simulink library "WECSim_Lib"  (R2014b)
settings: Solver=ode45  StartTime=0.0  StopTime=10.0  RelTol=1e-3
undefined symbols (not defined in the file): body, constraint, pto, simu, waves, X, Y, Z
libraries: nesl_utility x107, sm_lib x53
(part 4 of 4)

== system WECSim_Lib/Body Elements/Rigid Body/Wave Diffraction and Excitation Force Calculation/Linear Wave Excitation Force Variant Subsystem/Regular Wave Excitation Force ==
  note: Calculates the wave force, F_wave, for the case of Regular Waves.
      |
      | F_wave =   A * cos(w * t) * Re{Fext}
      |                -  A * sin(w * t) * Im{Fext}
  In1 : Inport
  Add : Sum
  Add1 : Sum  Inputs=+-
  Constant : Constant  Value=pi/2
  Excitation Imaginary Part : Constant  Value=body.hydroForce.fExt.im(1,:)  VectorParams1D=off
  Excitation Real Part : Constant  Value=body.hydroForce.fExt.re(1,:)  VectorParams1D=off
  Product : Product
  Product1 : Product  Inputs=3
  Product2 : Product  Inputs=3
  Sine Wave Function : Sin  TimeSource=Use external signal  SampleTime=0
  Sine Wave Function1 : Sin  TimeSource=Use external signal  SampleTime=0
  Wave Amplitude : Constant  Value=waves.A(1,:)
  Wave Frequency : Constant  Value=waves.w(1,:)
  Out1 : Outport
  wires:
  In1/1 -> Product/1  "t"
  Wave Frequency/1 -> Product/2  "w"
  Product/1 -> Sine Wave Function/1, Add/1
  Sine Wave Function1/1 -> Product1/3  "cos(w*t)"
  Sine Wave Function/1 -> Product2/2  "sin(wt)"
  Excitation Imaginary Part/1 -> Product2/3  "Im{Fext}"
  Excitation Real Part/1 -> Product1/2  "Re{Fext}"
  Product1/1 -> Add1/1
  Product2/1 -> Add1/2
  Add1/1 -> Out1/1
  Wave Amplitude/1 -> Product2/1, Product1/1  "A"
  Add/1 -> Sine Wave Function1/1
  Constant/1 -> Add/2

== system WECSim_Lib/Body Elements/Rigid Body/Wave Diffraction and Excitation Force Calculation/Linear Wave Excitation Force Variant Subsystem/User Defined Wave Excitation Force ==
  note: Calculates the wave force, F_wave, for the case of User Defined Waves.
      |
      | F_wave = convulation calculation [1x6]
  InputWaveForceTimeHistory : FromWorkspace  VariableName=[waves.waveAmpTime(:,1),body.hydroForce.userDefinedFe]  SampleTime=0
  Out1 : Outport
  wires:
  InputWaveForceTimeHistory/1 -> Out1/1

== system WECSim_Lib/Body Elements/Rigid Body/Wave Diffraction and Excitation Force Calculation/Nonlinear FK Force Variant Subsystem/No Nonlinear FroudeKrylov Force ==
  Constant : Constant  Value=[0 0 0 0 0 0]
  Out1 : Outport
  wires:
  Constant/1 -> Out1/1

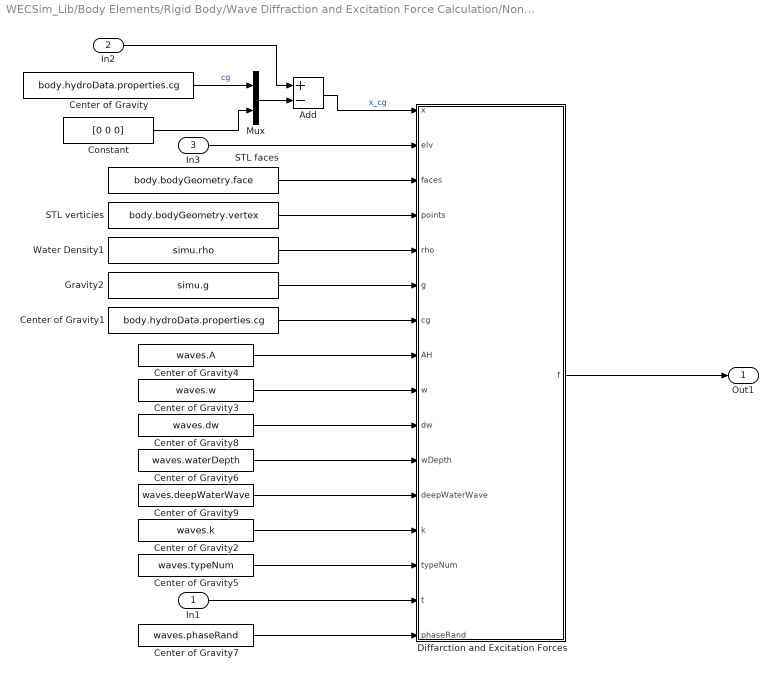
== system WECSim_Lib/Body Elements/Rigid Body/Wave Diffraction and Excitation Force Calculation/Nonlinear FK Force Variant Subsystem/With Nonlinear FroudeKrylov Force  ==
  In1 : Inport
  In2 : Inport  Port=2
  In3 : Inport  Port=3
  Add : Sum  Inputs=+-
  Center of Gravity : Constant  Value=body.hydroData.properties.cg
  Center of Gravity1 : Constant  Value=body.hydroData.properties.cg
  Center of Gravity2 : Constant  Value=waves.k
  Center of Gravity3 : Constant  Value=waves.w
  Center of Gravity4 : Constant  Value=waves.A
  Center of Gravity5 : Constant  Value=waves.typeNum
  Center of Gravity6 : Constant  Value=waves.waterDepth
  Center of Gravity7 : Constant  Value=waves.phaseRand
  Center of Gravity8 : Constant  Value=waves.dw
  Center of Gravity9 : Constant  Value=waves.deepWaterWave
  Constant : Constant  Value=[0 0 0]
  Diffarction and Excitation Forces : MATLAB Function  TreatAsAtomicUnit=on
  Gravity2 : Constant  Value=simu.g
  Mux : Mux  Inputs=2
  STL faces : Constant  Value=body.bodyGeometry.face
  STL verticies : Constant  Value=body.bodyGeometry.vertex
  Water Density1 : Constant  Value=simu.rho
  Out1 : Outport
  wires:
  Center of Gravity1/1 -> Diffarction and Excitation Forces/7(cg)
  Diffarction and Excitation Forces/1(f) -> Out1/1
  Gravity2/1 -> Diffarction and Excitation Forces/6(g)
  Water Density1/1 -> Diffarction and Excitation Forces/5(rho)
  STL verticies/1 -> Diffarction and Excitation Forces/4(points)
  STL faces/1 -> Diffarction and Excitation Forces/3(faces)
  In3/1 -> Diffarction and Excitation Forces/2(elv)
  In1/1 -> Diffarction and Excitation Forces/15(t)
  Center of Gravity4/1 -> Diffarction and Excitation Forces/8(AH)
  Center of Gravity3/1 -> Diffarction and Excitation Forces/9(w)
  Center of Gravity8/1 -> Diffarction and Excitation Forces/10(dw)
  Center of Gravity5/1 -> Diffarction and Excitation Forces/14(typeNum)
  Center of Gravity2/1 -> Diffarction and Excitation Forces/13(k)
  Center of Gravity6/1 -> Diffarction and Excitation Forces/11(wDepth)
  Center of Gravity7/1 -> Diffarction and Excitation Forces/16(phaseRand)
  Center of Gravity9/1 -> Diffarction and Excitation Forces/12(deepWaterWave)
  Add/1 -> Diffarction and Excitation Forces/1(x)  "x_cg"
  Mux/1 -> Add/2
  Center of Gravity/1 -> Mux/1  "cg"
  Constant/1 -> Mux/2
  In2/1 -> Add/1

== system WECSim_Lib/Body Elements/Rigid Body/Wave Radiation Forces Calculation/SS and CI Variant Subsystem/Converlution Integral Calculation ==
  In1 : Inport
  Fluid Memory1 : MATLAB Function  TreatAsAtomicUnit=on
  Impulse Response Function K1 : Constant  Value=body.hydroForce.irkb(:,1:6,1+(body.bodyNumber-1)*6:6+(body.bodyNumber-1)*6)
  Time (relative to the current time step)1 : Constant  Value=simu.CTTime
  Wave Type1 : Constant  Value=waves.typeNum
  Out1 : Outport
  wires:
  Wave Type1/1 -> Fluid Memory1/1(check)
  Time (relative to the current time step)1/1 -> Fluid Memory1/4(CTTime)
  Impulse Response Function K1/1 -> Fluid Memory1/3(IRKB)
  In1/1 -> Fluid Memory1/2(v)
  Fluid Memory1/1(F_FM) -> Out1/1  "F_Convolution Integral"

== system WECSim_Lib/Body Elements/Rigid Body/Wave Radiation Forces Calculation/SS and CI Variant Subsystem/State-Space Calculation  ==
  note: Calculates the net buoyancy and linear restoring forces
      | 	Net Buoyancy Force in z-direction = gravity force - buoyancy force = m*g - rho*g*Vol
      | 	Linear Restoring Force = linear restoring coefficient matrix * displacement about cg vector = k * x_cg
      |
      | For a floating body, the net boyancy force = 0.
  In1 : Inport
  State-Space : StateSpace  A=body.hydroForce.ssRadf.A  B=body.hydroForce.ssRadf.B  C=body.hydroForce.ssRadf.C  D=body.hydroForce.ssRadf.D  X0=0
  Out1 : Outport
  wires:
  State-Space/1 -> Out1/1
  In1/1 -> State-Space/1  "x"

== system WECSim_Lib/Body Elements/Rigid Body/Wave Diffraction and Excitation Force Calculation/Linear Wave Excitation Force Variant Subsystem/Irregular Wave Excitation Force/For Each Subsystem ==
  note: Calculates the Irregular wave force component for each individual frequency bin.
      |
      | F_wave(i) =  cos(w(i) * t + phi(i))  *  Re{Fext(i)}  *  sqrt(S(i) * dw)
      |                    - sin(w(i) * t + phi(i))  *  Im{Fext(i)}  *  sqrt(S(i) * dw)
  Wave Spectrum : Inport  Partition=on  PartitionDimension=1  PartitionWidth=1
  Wave Frequency : Inport  Port=2  Partition=on  PartitionDimension=1  PartitionWidth=1
  Real Part of Wave Excitation : Inport  Port=3  Partition=on  PartitionDimension=1  PartitionWidth=1
  Imaginary Part of Wave Excitation : Inport  Port=4  Partition=on  PartitionDimension=1  PartitionWidth=1
  Random Phase : Inport  Port=5  Partition=on  PartitionDimension=1  PartitionWidth=1
  Time : Inport  Port=6  Partition=off
  Add : Sum
  Add1 : Sum
  Add2 : Sum  Inputs=+-
  Constant1 : Constant  Value=pi/2
  For Each : ForEach  DisableCoverage=on  IndexMode=One-based
  Frequency Spacing Delta Omega : Constant  Value=waves.dw  VectorParams1D=off
  Product{,1..5} (6 alike) : Product  Inputs=**
  Sin Wave Function : Sin  TimeSource=Use external signal  SampleTime=0
  Sine Wave Function1 : Sin  TimeSource=Use external signal  SampleTime=0
  Sqrt : Sqrt  SaturateOnIntegerOverflow=on
  F_wave(i) : Outport  ConcatenationDimension=1
  wires:
  Add/1 -> Sin Wave Function/1, Add1/1
  Random Phase/1 -> Add/2  "phi(i)"
  Product1/1 -> Add/1
  Sqrt/1 -> Product3/1, Product2/2
  Product/1 -> Sqrt/1
  Frequency Spacing Delta Omega/1 -> Product/2  "dw"
  Wave Spectrum/1 -> Product/1  "S(i)"
  Time/1 -> Product1/2  "t"
  Add2/1 -> F_wave(i)/1
  Wave Frequency/1 -> Product1/1  "w(i)"
  Real Part of Wave Excitation/1 -> Product2/1  "Re{Fext(i)}"
  Imaginary Part of Wave Excitation/1 -> Product3/2  "Im{Fext(i)}"
  Product5/1 -> Add2/2
  Product4/1 -> Add2/1
  Product2/1 -> Product4/1  "Re{Fext(i)}  *  sqrt(S(i) * dw)"
  Product3/1 -> Product5/1  "Im{Fext(i)}  *  sqrt(S(i) * dw)"
  Sine Wave Function1/1 -> Product4/2  "cos(w(i) * t + phi(i))"
  Sin Wave Function/1 -> Product5/2  "sin(w(i) * t + phi(i))"
  Add1/1 -> Sine Wave Function1/1
  Constant1/1 -> Add1/2

== matlab function WECSim_Lib/Body Elements/Rigid Body/Wave Diffraction and Excitation Force Calculation/Nonlinear FK Force Variant Subsystem/With Nonlinear FroudeKrylov Force /Diffarction and Excitation Forces ==
  data: x input; elv input; faces input; f output; points input; rho input; g input; cg input; AH input; w input; dw input; wDepth input; deepWaterWave input; k input; typeNum input; t input; phaseRand input
function f  = nonFKForce(x,elv,faces,points,rho,g,cg,AH,w,dw,wDepth,deepWaterWave,k,typeNum,t,phaseRand)
% Function to calculate buoyancy force and moment on a triangulated surface
% NOTE: This function assumes that the STL file is imported with its CG at 0,0,0

% Compute new tri coords after cog rotation and translation
pointsMeanFS = offsetXYZ(points,cg);
centerMeanFS = triCenter(pointsMeanFS,faces);
avMeanFS     = triArea(pointsMeanFS,faces);

% Compute new tri coords after cog rotation and translation
points = rotateXYZ(points,[1 0 0],x(4));
points = rotateXYZ(points,[0 1 0],x(5));
points = rotateXYZ(points,[0 0 1],x(6));
points = offsetXYZ(points,x);
points = offsetXYZ(points,cg);

% Calculate new tri centers for hydrostatic pressure calc
center = triCenter(points,faces);

% Calculate tri area vectors, area, and normal vectors
av = triArea(points,faces);

% Calculate the free surface
wpMeanFS=pDis(centerMeanFS,       0,AH,w,dw,wDepth,deepWaterWave,t,k,phaseRand,typeNum,rho,g);
wp      =pDis(center      ,     elv,AH,w,dw,wDepth,deepWaterWave,t,k,phaseRand,typeNum,rho,g);

% Calculate the hydrostatic forces
f_linear   =FK(centerMeanFS,       cg,avMeanFS,wpMeanFS); %%% THIS WILL NEED TO HAVE THE CGR VECTOR ADDED WHEN ROTATION IS INCLUDED
f_nonLinear=FK(center      ,x(1:3)+cg,av      ,wp      ); %%% THIS WILL NEED TO HAVE THE CGR VECTOR ADDED WHEN ROTATION IS INCLUDED
f = f_nonLinear-f_linear;
end

function verts = offsetXYZ(verts,x)
% Function to move the position vertices
verts(:,1) = verts(:,1) + x(1);
verts(:,2) = verts(:,2) + x(2);
verts(:,3) = verts(:,3) + x(3);
end

function xn = rotateXYZ(x,ax,t)
% function to rotate a poitn about an arbitrary axis
% x: 3-componenet coordiantes
% ax: axis about which to rotate (must be a normal vector)
% t: rotation angle
% xn: new coordinates after rotation
rotMat = zeros(3);
rotMat(1,1) = ax(1)*ax(1)*(1-cos(t))    + cos(t);
rotMat(1,2) = ax(2)*ax(1)*(1-cos(t))    - ax(3)*sin(t);
rotMat(1,3) = ax(3)*ax(1)*(1-cos(t))    + ax(2)*sin(t);
rotMat(2,1) = ax(1)*ax(2)*(1-cos(t))    + ax(3)*sin(t);
rotMat(2,2) = ax(2)*ax(2)*(1-cos(t))    + cos(t);
rotMat(2,3) = ax(3)*ax(2)*(1-cos(t))    - ax(1)*sin(t);
rotMat(3,1) = ax(1)*ax(3)*(1-cos(t))    - ax(2)*sin(t);
rotMat(3,2) = ax(2)*ax(3)*(1-cos(t))    + ax(1)*sin(t);
rotMat(3,3) = ax(3)*ax(3)*(1-cos(t))    + cos(t);

xn = x*rotMat;
end

function c = triCenter(points,faces)
%Function to caculate the center coordinate of a triangle
% Inputs:
%     points: list of 3D points
%     faces: indicies that define the triangles
% Outputs:
%     c: centers of the triangles
c = zeros(length(faces),3);
c(:,1) = (points(faces(:,1),1)+points(faces(:,2),1)+points(faces(:,3),1))./3;
c(:,2) = (points(faces(:,1),2)+points(faces(:,2),2)+points(faces(:,3),2))./3;
c(:,3) = (points(faces(:,1),3)+points(faces(:,2),3)+points(faces(:,3),3))./3;
end

function av = triArea(points,faces)
% Function to calculate the area of a triangle
% Inputs:
%   p : points of the triangles
%   t : indicies of the points that make up triangles
% Outputs:
%   a: area of the triangles
%   nv: normal vector of the triangele
v1 = points(faces(:,3),:)-points(faces(:,1),:);
v2 = points(faces(:,2),:)-points(faces(:,1),:);
av =  1/2.*(cross(v1,v2));
end

function f=pDis(center,elv,AH,w,dw,wDepth,deepWaterWave,t,k,phaseRand,typeNum,rho,g)
f = zeros(length(center(:,3)),1);
if typeNum <10
elseif typeNum <20
    f = rho.*g.*AH(1).*cos(k(1).*center(:,1)-w(1)*t);
elseif typeNum <30
    tmp=sqrt(AH.*dw);
    tmp1 = ones(1,length(center(:,1)));
    tmp2 = (w.*t+phaseRand)*tmp1;
    tmp3 = cos(k*center(:,1)'- tmp2);
    f(:,1) = tmp3'*tmp.*rho.*g;
end
if deepWaterWave == 0
    z=(center(:,3)-elv).*wDepth./(wDepth+elv);
    f = f.*(cosh(k(1).*(z+wDepth))./cosh(k(1)*wDepth));
else
    z=(center(:,3)-elv);
    f = f.*exp(k.*z);
end
f(z>0)=0;
end

function f = FK(center,instcg,av,wp)
% Function to calculate the force and moment about the cog due to
% hydrostatic pressure
f = zeros(6,1);

% Calculate the hydrostatic pressure at each triangle center
pressureVect = [wp wp wp].*av;

% Compute force about cog
f(1:3) = sum(pressureVect);

% Compute moment about cog
tmp1 = ones(length(center(:,1)),1);
tmp2 = tmp1*instcg';
center2cgVec = center-tmp2;

f(4:6)= -sum(cross(center2cgVec,pressureVect));
end

== matlab function WECSim_Lib/Body Elements/Rigid Body/Wave Radiation Forces Calculation/SS and CI Variant Subsystem/Converlution Integral Calculation/Fluid Memory1 ==
  data: check input; v input; F_FM output; IRKB input; CTTime input
function F_FM = ConvolutionalIntegral(check,v,IRKB,CTTime)

%define persistent variables
persistent velocity;
persistent kkk
len = length(CTTime);

if check==10
    tmpT = zeros(6,1);
else
    if isempty(velocity)
        velocity = zeros(6,len);
        kkk=0;
    else
        kkk=kkk+1;
        int2=abs(kkk-floor(kkk/5)*5-1);
        if int2<0.00000001
            velocity(:,2:end) = velocity(:,1:end-1);
        end
        velocity(:,1) = v(:);
    end
    
    %integrate
    tmpT = zeros(6,1);
    for kd=1:6
        tmpV = zeros(len,1);
        for kk=1:6
            tmpY=IRKB(:,kd,kk).*velocity(kk,:)';
            tmpV = tmpV + tmpY;
        end
        tmpT(kd) = trapz(CTTime,tmpV);
    end
end
F_FM=tmpT;
end

== matlab function WECSim_Lib/Body Elements/Rigid Body/Nonlinear Wave Elevation/Linear or Instantaneous Free Surface/Instantaneous Water Free Surface  /Instantaneous FS ==
  data: x input; faces input; f output; points input; cg input; AH input; w input; dw input; k input; typeNum input; t input; rampT input; phaseRand input
function f  = waveElevation(x,faces,points,cg,AH,w,dw,k,typeNum,t,rampT,phaseRand)
% Function to calculate buoyancy force and moment on a triangulated surface
% NOTE: This function assumes that the STL file is imported with its CG at 0,0,0

% Compute new tri coords after cog rotation and translation
points = rotateXYZ(points,[1 0 0],x(4));
points = rotateXYZ(points,[0 1 0],x(5));
points = rotateXYZ(points,[0 0 1],x(6));
points = offsetXYZ(points,x);
points = offsetXYZ(points,cg);

% Calculate new tri centers for hydrostatic pressure calc
center = triCenter(points,faces);

% Calculate the free surface
f=waveElev(center,AH,w,dw,t,k,rampT,phaseRand,typeNum);

end

function verts = offsetXYZ(verts,x)
% Function to move the position vertices
verts(:,1) = verts(:,1) + x(1);
verts(:,2) = verts(:,2) + x(2);
verts(:,3) = verts(:,3) + x(3);
end

function xn = rotateXYZ(x,ax,t)
% function to rotate a poitn about an arbitrary axis
% x: 3-componenet coordiantes
% ax: axis about which to rotate (must be a normal vector)
% t: rotation angle
% xn: new coordinates after rotation
rotMat = zeros(3);
rotMat(1,1) = ax(1)*ax(1)*(1-cos(t))    + cos(t);
rotMat(1,2) = ax(2)*ax(1)*(1-cos(t))    - ax(3)*sin(t);
rotMat(1,3) = ax(3)*ax(1)*(1-cos(t))    + ax(2)*sin(t);
rotMat(2,1) = ax(1)*ax(2)*(1-cos(t))    + ax(3)*sin(t);
rotMat(2,2) = ax(2)*ax(2)*(1-cos(t))    + cos(t);
rotMat(2,3) = ax(3)*ax(2)*(1-cos(t))    - ax(1)*sin(t);
rotMat(3,1) = ax(1)*ax(3)*(1-cos(t))    - ax(2)*sin(t);
rotMat(3,2) = ax(2)*ax(3)*(1-cos(t))    + ax(1)*sin(t);
rotMat(3,3) = ax(3)*ax(3)*(1-cos(t))    + cos(t);

xn = x*rotMat;
end

function c = triCenter(points,faces)
%Function to caculate the center coordinate of a triangle
% Inputs:
%     points: list of 3D points
%     faces: indicies that define the triangles
% Outputs:
%     c: centers of the triangles
c = zeros(length(faces),3);
c(:,1) = (points(faces(:,1),1)+points(faces(:,2),1)+points(faces(:,3),1))./3;
c(:,2) = (points(faces(:,1),2)+points(faces(:,2),2)+points(faces(:,3),2))./3;
c(:,3) = (points(faces(:,1),3)+points(faces(:,2),3)+points(faces(:,3),3))./3;
end

function f=waveElev(center,AH,w,dw,t,k,rampT,phaseRand,typeNum)
f = zeros(length(center(:,3)),1);
if typeNum <10
elseif typeNum <20
    f = AH(1).*cos(k(1).*center(:,1)-w(1)*t);
elseif typeNum <30
    tmp=sqrt(AH.*dw);
    tmp1 = ones(1,length(center(:,1)));
    tmp2 = (w.*t+phaseRand)*tmp1;
    tmp3 = cos(k*center(:,1)'- tmp2);
    f(:,1) = tmp3'*tmp;
end
if t<=rampT
    rampF = (1+cos(pi+pi*t/rampT))/2;
    f = f.*rampF;
end

end

== matlab function WECSim_Lib/Body Elements/Rigid Body/Hydrostatic Restoring Force Calculation/Linear and Nonlinear Restoring Force Variant Subsystem/Nonlinear Hydrostatic Restoring Force /Diffarction and Excitation Forces1 ==
  data: x input; elv input; faces input; f output; points input; rho input; g input; cg input
function f  = nonLinearBuoyancy(x,elv,faces,points,rho,g,cg)
% Function to calculate buoyancy force and moment on a triangulated surface
% NOTE: This function assumes that the STL file is imported with its CG at 0,0,0

% Compute new tri coords after cog rotation and translation
points = rotateXYZ(points,[1 0 0],x(4));
points = rotateXYZ(points,[0 1 0],x(5));
points = rotateXYZ(points,[0 0 1],x(6));
points = offsetXYZ(points,x);
points = offsetXYZ(points,cg);

% Calculate new tri centers for hydrostatic pressure calc
center = triCenter(points,faces);

% Calculate tri area vectors, area, and normal vectors
av = triArea(points,faces);

% Calculate the hydrostatic forces
f=fHydrostatic(center,elv,x(1:3)+cg,av,rho,g); %%% THIS WILL NEED TO HAVE THE CGR VECTOR ADDED WHEN ROTATION IS INCLUDED
end

function verts = offsetXYZ(verts,x)
% Function to move the position vertices
verts(:,1) = verts(:,1) + x(1);
verts(:,2) = verts(:,2) + x(2);
verts(:,3) = verts(:,3) + x(3);
end

function xn = rotateXYZ(x,ax,t)
% function to rotate a poitn about an arbitrary axis
% x: 3-componenet coordiantes
% ax: axis about which to rotate (must be a normal vector)
% t: rotation angle
% xn: new coordinates after rotation
rotMat = zeros(3);
rotMat(1,1) = ax(1)*ax(1)*(1-cos(t))    + cos(t);
rotMat(1,2) = ax(2)*ax(1)*(1-cos(t))    - ax(3)*sin(t);
rotMat(1,3) = ax(3)*ax(1)*(1-cos(t))    + ax(2)*sin(t);
rotMat(2,1) = ax(1)*ax(2)*(1-cos(t))    + ax(3)*sin(t);
rotMat(2,2) = ax(2)*ax(2)*(1-cos(t))    + cos(t);
rotMat(2,3) = ax(3)*ax(2)*(1-cos(t))    - ax(1)*sin(t);
rotMat(3,1) = ax(1)*ax(3)*(1-cos(t))    - ax(2)*sin(t);
rotMat(3,2) = ax(2)*ax(3)*(1-cos(t))    + ax(1)*sin(t);
rotMat(3,3) = ax(3)*ax(3)*(1-cos(t))    + cos(t);

xn = x*rotMat;
end

function c = triCenter(points,faces)
%Function to caculate the center coordinate of a triangle
% Inputs:
%     points: list of 3D points
%     faces: indicies that define the triangles
% Outputs:
%     c: centers of the triangles
c = zeros(length(faces),3);
c(:,1) = (points(faces(:,1),1)+points(faces(:,2),1)+points(faces(:,3),1))./3;
c(:,2) = (points(faces(:,1),2)+points(faces(:,2),2)+points(faces(:,3),2))./3;
c(:,3) = (points(faces(:,1),3)+points(faces(:,2),3)+points(faces(:,3),3))./3;
end

function av = triArea(points,faces)
% Function to calculate the area of a triangle
% Inputs:
%   p : points of the triangles
%   t : indicies of the points that make up triangles
% Outputs:
%   a: area of the triangles
%   nv: normal vector of the triangele
v1 = points(faces(:,3),:)-points(faces(:,1),:);
v2 = points(faces(:,2),:)-points(faces(:,1),:);
av =  1/2.*(cross(v1,v2));
end

function f = fHydrostatic(center,elv,instcg,av,rho,g)
% Function to calculate the force and moment about the cog due to
% hydrostatic pressure
f = zeros(6,1);

% Zeor out regions above the mean free surface
z=center(:,3); z((z-elv)>0)=0;

% Calculate the hydrostatic pressure at each triangle center
pressureVect = rho*g.*[-z -z -z].*av;

% Compute force about cog
f(1:3) = sum(pressureVect);

tmp1 = ones(length(center(:,1)),1);
tmp2 = tmp1*instcg';
center2cgVec = center-tmp2;

f(4:6)= -sum(cross(center2cgVec,pressureVect));
end

== matlab function WECSim_Lib/Body Elements/Rigid Body/Structure/Motion Sensor/Angle ==
  data: Q input; E output
function E  = EulerAngle(Q)
%#codegen
E=zeros(3,1);
E(1) = atan2( (2*(Q(1)*Q(2)+Q(3)*Q(4))), (1-2* (Q(2)^2+Q(3)^2) ) );
E(2) = asin( 2* (Q(1)*Q(3) - Q(4)*Q(2)));
E(3) = atan2( (2*(Q(1)*Q(4)+Q(2)*Q(3))), (1-2* (Q(3)^2+Q(4)^2) ) );
